simulink model "Attitude_Control_Pyramidal_Configuration"  (R2024b)
settings: Solver=VariableStepAuto  StartTime=0.0  StopTime=10.0  RelTol=1e-3
libraries: slpidlib x7, simulink_extras x1, matrix_library x1, aerolibutil x1
settings Model: Creator=LEGION  LastModifiedBy=LEGION
settings DebuggingCC: AlgebraicLoopMsg=none

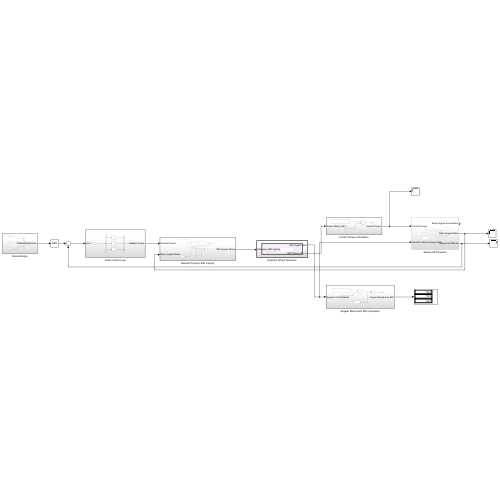
[thumbnail: Simulink's stored preview of the top-level diagram]
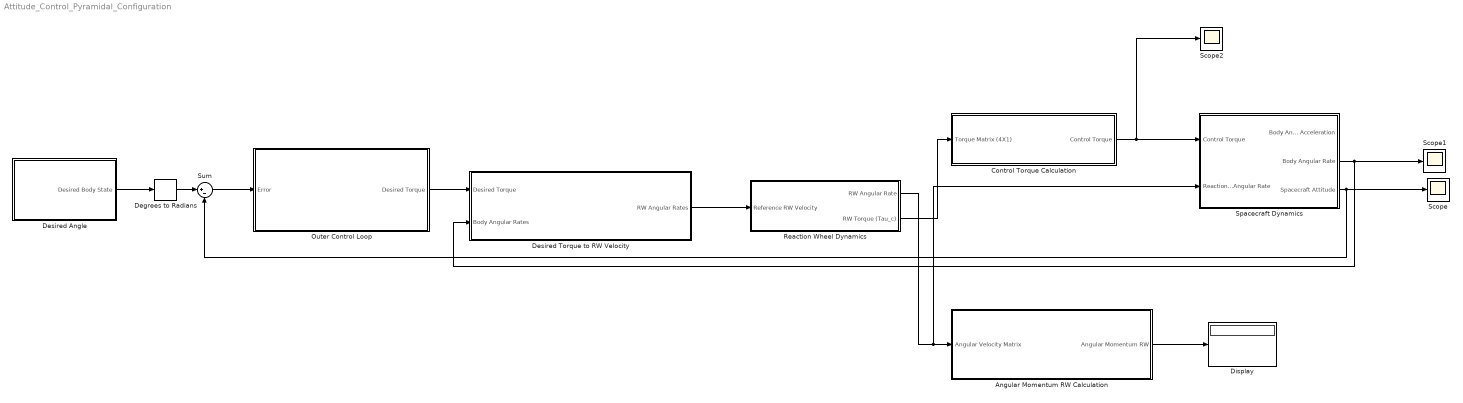
== system Attitude_Control_Pyramidal_Configuration ==
  Angular Momentum RW Calculation : Subsystem
  Control Torque Calculation : Subsystem
  Degrees to Radians : simulink_extras/Transformations/Degrees to Radians
  Desired Angle : Subsystem
  Desired Torque to RW Velocity : Subsystem
  Display : Display
  Outer Control Loop : Subsystem
  Reaction Wheel Dynamics : Subsystem  TreatAsAtomicUnit=on
      settings: MinAlgLoopOccurrences=on
  Scope : Scope
  Scope1 : Scope
  Scope2 : Scope
  Spacecraft Dynamics : Subsystem
      settings: PermitHierarchicalResolution=None  MinAlgLoopOccurrences=on
  Sum : Sum  Inputs=|+-
  wires:
  Control Torque Calculation/1(Control Torque) -> Scope2/1, Spacecraft Dynamics/1(Control Torque)
  Desired Angle/1(Desired Body State) -> Degrees to Radians/1
  Degrees to Radians/1 -> Sum/1
  Sum/1 -> Outer Control Loop/1(Error)
  Outer Control Loop/1(Desired Torque) -> Desired Torque to RW Velocity/1(Desired Torque)
  Reaction Wheel Dynamics/1(RW Angular Rate) -> Spacecraft Dynamics/2(Reaction Wheel Angular Rate), Angular Momentum RW Calculation/1("Angular Velocity Matrix ")
  Reaction Wheel Dynamics/2(RW Torque (Tau_c)) -> Control Torque Calculation/1(Torque Matrix (4X1))
  Desired Torque to RW Velocity/1(RW Angular Rates) -> Reaction Wheel Dynamics/1(Reference RW Velocity)
  Spacecraft Dynamics/2(Body Angular Rate) -> Scope1/1, Desired Torque to RW Velocity/2(Body Angular Rates)
  Spacecraft Dynamics/3(Spacecraft Attitude) -> Scope/1, Sum/2
  Angular Momentum RW Calculation/1(Angular Momentum RW) -> Display/1

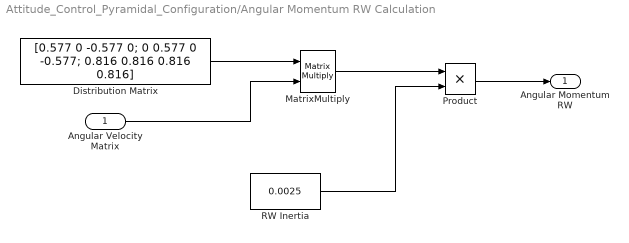
== system Attitude_Control_Pyramidal_Configuration/Angular Momentum RW Calculation ==
  "Angular Velocity Matrix " : Inport
  Distribution Matrix : Constant  Value=[0.577 0 -0.577 0; 0 0.577 0 -0.577; 0.816 0.816 0.816 0.816]  VectorParams1D=off
  MatrixMultiply : Product  Multiplication=Matrix(*)
  Product : Product
  RW Inertia : Constant  Value=0.0025
  Angular Momentum RW : Outport
  wires:
  Distribution Matrix/1 -> MatrixMultiply/1
  "Angular Velocity Matrix "/1 -> MatrixMultiply/2
  MatrixMultiply/1 -> Product/1
  RW Inertia/1 -> Product/2
  Product/1 -> Angular Momentum RW/1

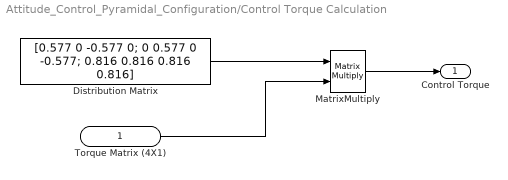
== system Attitude_Control_Pyramidal_Configuration/Control Torque Calculation ==
  Torque Matrix (4X1) : Inport
  Distribution Matrix : Constant  Value=[0.577 0 -0.577 0; 0 0.577 0 -0.577; 0.816 0.816 0.816 0.816]  VectorParams1D=off
  MatrixMultiply : Product  Multiplication=Matrix(*)
  Control Torque : Outport
  wires:
  Distribution Matrix/1 -> MatrixMultiply/1
  Torque Matrix (4X1)/1 -> MatrixMultiply/2
  MatrixMultiply/1 -> Control Torque/1

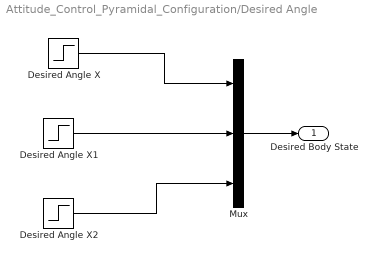
== system Attitude_Control_Pyramidal_Configuration/Desired Angle ==
  Desired Angle X : Step  Time=0.1  After=90  SampleTime=0  VectorParams1D=off
  Desired Angle X1 : Step  Time=0.1  After=90  SampleTime=0  VectorParams1D=off
  Desired Angle X2 : Step  Time=0.1  After=90  SampleTime=0  VectorParams1D=off
  Mux : Mux  Inputs=3
  Desired Body State : Outport
  wires:
  Desired Angle X1/1 -> Mux/2
  Desired Angle X/1 -> Mux/1
  Desired Angle X2/1 -> Mux/3
  Mux/1 -> Desired Body State/1

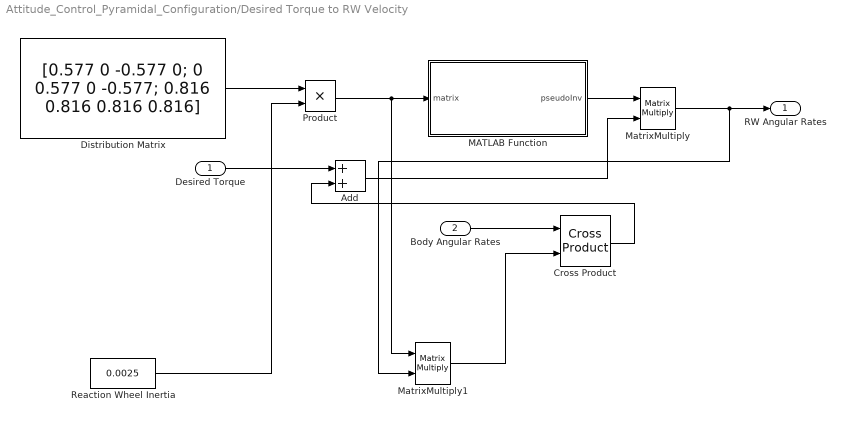
== system Attitude_Control_Pyramidal_Configuration/Desired Torque to RW Velocity ==
  Desired Torque : Inport
  Body Angular Rates : Inport  Port=2
  Add : Sum
  Cross Product : matrix_library/Cross Product
  Distribution Matrix : Constant  Value=[0.577 0 -0.577 0; 0 0.577 0 -0.577; 0.816 0.816 0.816 0.816]  VectorParams1D=off
  MATLAB Function : MATLAB Function  TreatAsAtomicUnit=on
  MatrixMultiply : Product  Multiplication=Matrix(*)
  MatrixMultiply1 : Product  Multiplication=Matrix(*)
  Product : Product
  Reaction Wheel Inertia : Constant  Value=0.0025
  RW Angular Rates : Outport
  wires:
  Desired Torque/1 -> Add/1
  Distribution Matrix/1 -> Product/1
  Reaction Wheel Inertia/1 -> Product/2
  Product/1 -> MATLAB Function/1(matrix), MatrixMultiply1/1
  MATLAB Function/1(pseudoInv) -> MatrixMultiply/1
  Body Angular Rates/1 -> Cross Product/1
  Cross Product/1 -> Add/2
  Add/1 -> MatrixMultiply/2
  MatrixMultiply/1 -> MatrixMultiply1/2, RW Angular Rates/1
  MatrixMultiply1/1 -> Cross Product/2

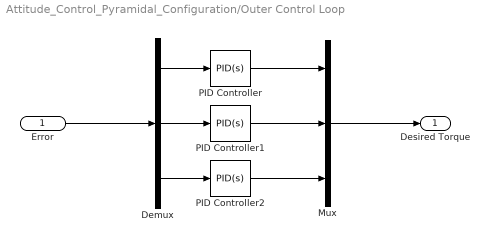
== system Attitude_Control_Pyramidal_Configuration/Outer Control Loop ==
  Error : Inport
  Demux : Demux  Outputs=3
  Mux : Mux  Inputs=3
  PID Controller : slpidlib/PID Controller  Controller=PID  Form=Parallel  TimeDomain=Continuous-time  UseExternalTs=off  SampleTime=-1  IntegratorMethod=Forward Euler  FilterMethod=Forward Euler  ControllerParametersSource=internal  P=100  I=1  UseKiTs=off  D=5  UseExternalDerivativeSource=off  N=100  UseFilter=on  TunerSelectOption=Transfer Function Based (PID Tuner App)  InitialConditionSource=internal  InitialConditionForIntegrator=0  InitialConditionForFilter=0  DifferentiatorICPrevScaledInput=0  ExternalReset=none  TrackingMode=off  Kt=1  LimitOutput=off  SatLimitsSource=internal  UpperSaturationLimit=inf  LowerSaturationLimit=-inf  LinearizeAsGain=on  AntiWindupMode=none  Kb=1  LimitIntegrator=off  UpperIntegratorSaturationLimit=inf  LowerIntegratorSaturationLimit=-inf  POutMin=[]  POutMax=[]  IOutMin=[]  IOutMax=[]  DOutMin=[]  DOutMax=[]  NOutMin=[]  NOutMax=[]  SumOutMin=[]  SumOutMax=[]  SaturationOutMin=[]  SaturationOutMax=[]  PParamMin=[]  PParamMax=[]  IParamMin=[]  IParamMax=[]  DParamMin=[]  DParamMax=[]  NParamMin=[]  NParamMax=[]  KbParamMin=[]  KbParamMax=[]  KtParamMin=[]  KtParamMax=[]  KbOutMin=[]  KbOutMax=[]  KtOutMin=[]  KtOutMax=[]  IntegratorOutMin=[]  IntegratorOutMax=[]  FilterOutMin=[]  FilterOutMax=[]  SumI1OutMin=[]  SumI1OutMax=[]  SumI2OutMin=[]  SumI2OutMax=[]  SumI3OutMin=[]  SumI3OutMax=[]  SumI4OutMin=[]  SumI4OutMax=[]  SumDOutMin=[]  SumDOutMax=[]  DifferentiatorOutMin=[]  DifferentiatorOutMax=[]  FilterDiffOutCoefMin=[]  FilterDiffOutCoefMax=[]  ReciprocalOutMin=[]  ReciprocalOutMax=[]  SumDenOutMin=[]  SumDenOutMax=[]  SumNumOutMin=[]  SumNumOutMax=[]  DivideOutMin=[]  DivideOutMax=[]  UdiffTsProdOutMin=[]  UdiffTsProdOutMax=[]  NTsProdOutMin=[]  NTsProdOutMax=[]  UintegralTsProdOutMin=[]  UintegralTsProdOutMax=[]  UngainTsProdOutMin=[]  UngainTsProdOutMax=[]  ClampingZeroOutDataTypeStr=Inherit: Inherit via back propagation  ClampingZeroOutMin=[]  ClampingZeroOutMax=[]  FilterDenConstantOutDataTypeStr=Inherit: Inherit via back propagation  FilterDenConstantOutMin=[]  FilterDenConstantOutMax=[]  PCopyOutDataTypeStr=Inherit: Inherit via back propagation  PCopyOutMin=[]  PCopyOutMax=[]  NCopyOutDataTypeStr=Inherit: Inherit via back propagation  NCopyOutMin=[]  NCopyOutMax=[]  IntegratorContinuousStateAttributes=''  IntegratorStateMustResolveToSignalObject=off  IntegratorRTWStateStorageClass=Auto  FilterContinuousStateAttributes=''  FilterStateMustResolveToSignalObject=off  FilterRTWStateStorageClass=Auto  ParallelPVariant=InternalParameters  IdealPVariant=Disabled  IVariant=InternalParameters  DVariant=InternalParameters  IntegratorVariant=Continuous  SatVariant=Disabled  AWVariant=Passthrough  PCopyVariant=Disabled  TRVariant=Disabled  FdbkBlocksVariant=Forward  IdealPFdbkVariant=Disabled  SatFdbkVariant=Disabled  DerivativeFilterVariant=ContFilter  NVariant=InternalParameters  NCopyVariant=Disabled  FilterICVariant=InternalICsFilter  IntegratorICVariant=InternalICs  ExternalResetVariant=Disabled  TRSumVariant=Passthrough  SumFdbkVariant=Disabled  SumVariant=Sum_PID  TsampFilterVariant=InternalTs  TsampNgainVariant=Passthrough  TsampIntegralVariant=Disabled_SignalSpec  ExternalSaturationOutDataTypeStr=Inherit: Same as second input  DerivativeSourceVariant=ErrorSignal  PreIntVariant=InternalPreInt
  PID Controller1 : slpidlib/PID Controller  Controller=PID  Form=Parallel  TimeDomain=Continuous-time  UseExternalTs=off  SampleTime=-1  IntegratorMethod=Forward Euler  FilterMethod=Forward Euler  ControllerParametersSource=internal  P=100  I=1  UseKiTs=off  D=5  UseExternalDerivativeSource=off  N=100  UseFilter=on  TunerSelectOption=Transfer Function Based (PID Tuner App)  InitialConditionSource=internal  InitialConditionForIntegrator=0  InitialConditionForFilter=0  DifferentiatorICPrevScaledInput=0  ExternalReset=none  TrackingMode=off  Kt=1  LimitOutput=off  SatLimitsSource=internal  UpperSaturationLimit=inf  LowerSaturationLimit=-inf  LinearizeAsGain=on  AntiWindupMode=none  Kb=1  LimitIntegrator=off  UpperIntegratorSaturationLimit=inf  LowerIntegratorSaturationLimit=-inf  POutMin=[]  POutMax=[]  IOutMin=[]  IOutMax=[]  DOutMin=[]  DOutMax=[]  NOutMin=[]  NOutMax=[]  SumOutMin=[]  SumOutMax=[]  SaturationOutMin=[]  SaturationOutMax=[]  PParamMin=[]  PParamMax=[]  IParamMin=[]  IParamMax=[]  DParamMin=[]  DParamMax=[]  NParamMin=[]  NParamMax=[]  KbParamMin=[]  KbParamMax=[]  KtParamMin=[]  KtParamMax=[]  KbOutMin=[]  KbOutMax=[]  KtOutMin=[]  KtOutMax=[]  IntegratorOutMin=[]  IntegratorOutMax=[]  FilterOutMin=[]  FilterOutMax=[]  SumI1OutMin=[]  SumI1OutMax=[]  SumI2OutMin=[]  SumI2OutMax=[]  SumI3OutMin=[]  SumI3OutMax=[]  SumI4OutMin=[]  SumI4OutMax=[]  SumDOutMin=[]  SumDOutMax=[]  DifferentiatorOutMin=[]  DifferentiatorOutMax=[]  FilterDiffOutCoefMin=[]  FilterDiffOutCoefMax=[]  ReciprocalOutMin=[]  ReciprocalOutMax=[]  SumDenOutMin=[]  SumDenOutMax=[]  SumNumOutMin=[]  SumNumOutMax=[]  DivideOutMin=[]  DivideOutMax=[]  UdiffTsProdOutMin=[]  UdiffTsProdOutMax=[]  NTsProdOutMin=[]  NTsProdOutMax=[]  UintegralTsProdOutMin=[]  UintegralTsProdOutMax=[]  UngainTsProdOutMin=[]  UngainTsProdOutMax=[]  ClampingZeroOutDataTypeStr=Inherit: Inherit via back propagation  ClampingZeroOutMin=[]  ClampingZeroOutMax=[]  FilterDenConstantOutDataTypeStr=Inherit: Inherit via back propagation  FilterDenConstantOutMin=[]  FilterDenConstantOutMax=[]  PCopyOutDataTypeStr=Inherit: Inherit via back propagation  PCopyOutMin=[]  PCopyOutMax=[]  NCopyOutDataTypeStr=Inherit: Inherit via back propagation  NCopyOutMin=[]  NCopyOutMax=[]  IntegratorContinuousStateAttributes=''  IntegratorStateMustResolveToSignalObject=off  IntegratorRTWStateStorageClass=Auto  FilterContinuousStateAttributes=''  FilterStateMustResolveToSignalObject=off  FilterRTWStateStorageClass=Auto  ParallelPVariant=InternalParameters  IdealPVariant=Disabled  IVariant=InternalParameters  DVariant=InternalParameters  IntegratorVariant=Continuous  SatVariant=Disabled  AWVariant=Passthrough  PCopyVariant=Disabled  TRVariant=Disabled  FdbkBlocksVariant=Forward  IdealPFdbkVariant=Disabled  SatFdbkVariant=Disabled  DerivativeFilterVariant=ContFilter  NVariant=InternalParameters  NCopyVariant=Disabled  FilterICVariant=InternalICsFilter  IntegratorICVariant=InternalICs  ExternalResetVariant=Disabled  TRSumVariant=Passthrough  SumFdbkVariant=Disabled  SumVariant=Sum_PID  TsampFilterVariant=InternalTs  TsampNgainVariant=Passthrough  TsampIntegralVariant=Disabled_SignalSpec  ExternalSaturationOutDataTypeStr=Inherit: Same as second input  DerivativeSourceVariant=ErrorSignal  PreIntVariant=InternalPreInt
  PID Controller2 : slpidlib/PID Controller  Controller=PID  Form=Parallel  TimeDomain=Continuous-time  UseExternalTs=off  SampleTime=-1  IntegratorMethod=Forward Euler  FilterMethod=Forward Euler  ControllerParametersSource=internal  P=100  I=1  UseKiTs=off  D=5  UseExternalDerivativeSource=off  N=100  UseFilter=on  TunerSelectOption=Transfer Function Based (PID Tuner App)  InitialConditionSource=internal  InitialConditionForIntegrator=0  InitialConditionForFilter=0  DifferentiatorICPrevScaledInput=0  ExternalReset=none  TrackingMode=off  Kt=1  LimitOutput=off  SatLimitsSource=internal  UpperSaturationLimit=inf  LowerSaturationLimit=-inf  LinearizeAsGain=on  AntiWindupMode=none  Kb=1  LimitIntegrator=off  UpperIntegratorSaturationLimit=inf  LowerIntegratorSaturationLimit=-inf  POutMin=[]  POutMax=[]  IOutMin=[]  IOutMax=[]  DOutMin=[]  DOutMax=[]  NOutMin=[]  NOutMax=[]  SumOutMin=[]  SumOutMax=[]  SaturationOutMin=[]  SaturationOutMax=[]  PParamMin=[]  PParamMax=[]  IParamMin=[]  IParamMax=[]  DParamMin=[]  DParamMax=[]  NParamMin=[]  NParamMax=[]  KbParamMin=[]  KbParamMax=[]  KtParamMin=[]  KtParamMax=[]  KbOutMin=[]  KbOutMax=[]  KtOutMin=[]  KtOutMax=[]  IntegratorOutMin=[]  IntegratorOutMax=[]  FilterOutMin=[]  FilterOutMax=[]  SumI1OutMin=[]  SumI1OutMax=[]  SumI2OutMin=[]  SumI2OutMax=[]  SumI3OutMin=[]  SumI3OutMax=[]  SumI4OutMin=[]  SumI4OutMax=[]  SumDOutMin=[]  SumDOutMax=[]  DifferentiatorOutMin=[]  DifferentiatorOutMax=[]  FilterDiffOutCoefMin=[]  FilterDiffOutCoefMax=[]  ReciprocalOutMin=[]  ReciprocalOutMax=[]  SumDenOutMin=[]  SumDenOutMax=[]  SumNumOutMin=[]  SumNumOutMax=[]  DivideOutMin=[]  DivideOutMax=[]  UdiffTsProdOutMin=[]  UdiffTsProdOutMax=[]  NTsProdOutMin=[]  NTsProdOutMax=[]  UintegralTsProdOutMin=[]  UintegralTsProdOutMax=[]  UngainTsProdOutMin=[]  UngainTsProdOutMax=[]  ClampingZeroOutDataTypeStr=Inherit: Inherit via back propagation  ClampingZeroOutMin=[]  ClampingZeroOutMax=[]  FilterDenConstantOutDataTypeStr=Inherit: Inherit via back propagation  FilterDenConstantOutMin=[]  FilterDenConstantOutMax=[]  PCopyOutDataTypeStr=Inherit: Inherit via back propagation  PCopyOutMin=[]  PCopyOutMax=[]  NCopyOutDataTypeStr=Inherit: Inherit via back propagation  NCopyOutMin=[]  NCopyOutMax=[]  IntegratorContinuousStateAttributes=''  IntegratorStateMustResolveToSignalObject=off  IntegratorRTWStateStorageClass=Auto  FilterContinuousStateAttributes=''  FilterStateMustResolveToSignalObject=off  FilterRTWStateStorageClass=Auto  ParallelPVariant=InternalParameters  IdealPVariant=Disabled  IVariant=InternalParameters  DVariant=InternalParameters  IntegratorVariant=Continuous  SatVariant=Disabled  AWVariant=Passthrough  PCopyVariant=Disabled  TRVariant=Disabled  FdbkBlocksVariant=Forward  IdealPFdbkVariant=Disabled  SatFdbkVariant=Disabled  DerivativeFilterVariant=ContFilter  NVariant=InternalParameters  NCopyVariant=Disabled  FilterICVariant=InternalICsFilter  IntegratorICVariant=InternalICs  ExternalResetVariant=Disabled  TRSumVariant=Passthrough  SumFdbkVariant=Disabled  SumVariant=Sum_PID  TsampFilterVariant=InternalTs  TsampNgainVariant=Passthrough  TsampIntegralVariant=Disabled_SignalSpec  ExternalSaturationOutDataTypeStr=Inherit: Same as second input  DerivativeSourceVariant=ErrorSignal  PreIntVariant=InternalPreInt
  Desired Torque : Outport
  wires:
  Error/1 -> Demux/1
  Demux/1 -> PID Controller/1
  Demux/2 -> PID Controller1/1
  Demux/3 -> PID Controller2/1
  PID Controller/1 -> Mux/1
  PID Controller1/1 -> Mux/2
  PID Controller2/1 -> Mux/3
  Mux/1 -> Desired Torque/1

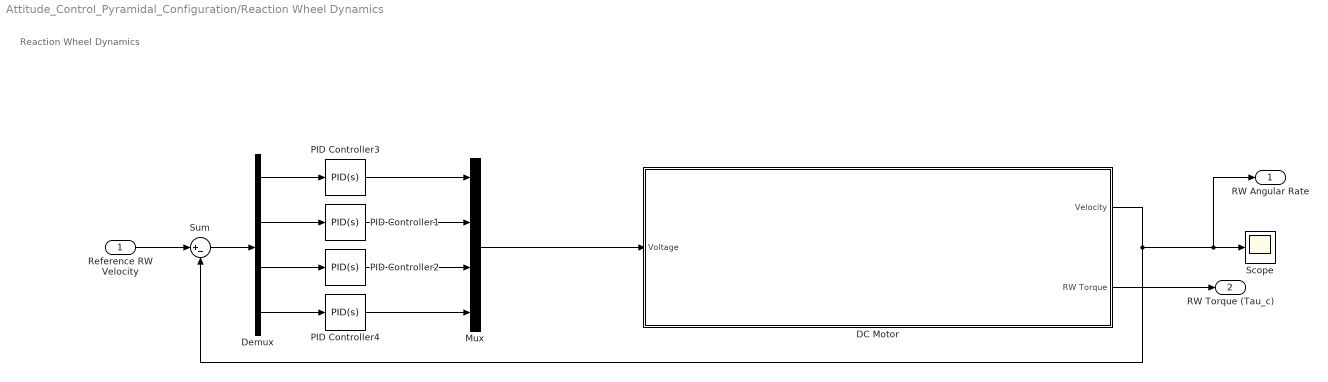
== system Attitude_Control_Pyramidal_Configuration/Reaction Wheel Dynamics ==
  note: Reaction Wheel Dynamics
  Reference RW Velocity : Inport
  "DC Motor " : Subsystem
  Demux : Demux
  Mux : Mux
  PID Controller{1..4} (4 alike) : slpidlib/PID Controller  Controller=PID  Form=Parallel  TimeDomain=Continuous-time  UseExternalTs=off  SampleTime=-1  IntegratorMethod=Forward Euler  FilterMethod=Forward Euler  ControllerParametersSource=internal  P=0.0171217142145511  I=12.0565982426295  UseKiTs=off  D=0  UseExternalDerivativeSource=off  N=100  UseFilter=on  TunerSelectOption=Transfer Function Based (PID Tuner App)  InitialConditionSource=internal  InitialConditionForIntegrator=0  InitialConditionForFilter=0  DifferentiatorICPrevScaledInput=0  ExternalReset=none  TrackingMode=off  Kt=1  LimitOutput=off  SatLimitsSource=internal  UpperSaturationLimit=inf  LowerSaturationLimit=-inf  LinearizeAsGain=on  AntiWindupMode=none  Kb=1  LimitIntegrator=off  UpperIntegratorSaturationLimit=inf  LowerIntegratorSaturationLimit=-inf  POutMin=[]  POutMax=[]  IOutMin=[]  IOutMax=[]  DOutMin=[]  DOutMax=[]  NOutMin=[]  NOutMax=[]  SumOutMin=[]  SumOutMax=[]  SaturationOutMin=[]  SaturationOutMax=[]  PParamMin=[]  PParamMax=[]  IParamMin=[]  IParamMax=[]  DParamMin=[]  DParamMax=[]  NParamMin=[]  NParamMax=[]  KbParamMin=[]  KbParamMax=[]  KtParamMin=[]  KtParamMax=[]  KbOutMin=[]  KbOutMax=[]  KtOutMin=[]  KtOutMax=[]  IntegratorOutMin=[]  IntegratorOutMax=[]  FilterOutMin=[]  FilterOutMax=[]  SumI1OutMin=[]  SumI1OutMax=[]  SumI2OutMin=[]  SumI2OutMax=[]  SumI3OutMin=[]  SumI3OutMax=[]  SumI4OutMin=[]  SumI4OutMax=[]  SumDOutMin=[]  SumDOutMax=[]  DifferentiatorOutMin=[]  DifferentiatorOutMax=[]  FilterDiffOutCoefMin=[]  FilterDiffOutCoefMax=[]  ReciprocalOutMin=[]  ReciprocalOutMax=[]  SumDenOutMin=[]  SumDenOutMax=[]  SumNumOutMin=[]  SumNumOutMax=[]  DivideOutMin=[]  DivideOutMax=[]  UdiffTsProdOutMin=[]  UdiffTsProdOutMax=[]  NTsProdOutMin=[]  NTsProdOutMax=[]  UintegralTsProdOutMin=[]  UintegralTsProdOutMax=[]  UngainTsProdOutMin=[]  UngainTsProdOutMax=[]  ClampingZeroOutDataTypeStr=Inherit: Inherit via back propagation  ClampingZeroOutMin=[]  ClampingZeroOutMax=[]  FilterDenConstantOutDataTypeStr=Inherit: Inherit via back propagation  FilterDenConstantOutMin=[]  FilterDenConstantOutMax=[]  PCopyOutDataTypeStr=Inherit: Inherit via back propagation  PCopyOutMin=[]  PCopyOutMax=[]  NCopyOutDataTypeStr=Inherit: Inherit via back propagation  NCopyOutMin=[]  NCopyOutMax=[]  IntegratorContinuousStateAttributes=''  IntegratorStateMustResolveToSignalObject=off  IntegratorRTWStateStorageClass=Auto  FilterContinuousStateAttributes=''  FilterStateMustResolveToSignalObject=off  FilterRTWStateStorageClass=Auto  ParallelPVariant=InternalParameters  IdealPVariant=Disabled  IVariant=InternalParameters  DVariant=InternalParameters  IntegratorVariant=Continuous  SatVariant=Disabled  AWVariant=Passthrough  PCopyVariant=Disabled  TRVariant=Disabled  FdbkBlocksVariant=Forward  IdealPFdbkVariant=Disabled  SatFdbkVariant=Disabled  DerivativeFilterVariant=ContFilter  NVariant=InternalParameters  NCopyVariant=Disabled  FilterICVariant=InternalICsFilter  IntegratorICVariant=InternalICs  ExternalResetVariant=Disabled  TRSumVariant=Passthrough  SumFdbkVariant=Disabled  SumVariant=Sum_PID  TsampFilterVariant=InternalTs  TsampNgainVariant=Passthrough  TsampIntegralVariant=Disabled_SignalSpec  ExternalSaturationOutDataTypeStr=Inherit: Same as second input  DerivativeSourceVariant=ErrorSignal  PreIntVariant=InternalPreInt
  Scope : Scope
  Sum : Sum  Inputs=|+-
  RW Angular Rate : Outport
  RW Torque (Tau_c) : Outport  Port=2
  wires:
  "DC Motor "/1(Velocity) -> Sum/2, RW Angular Rate/1, Scope/1
  Sum/1 -> Demux/1
  Demux/1 -> PID Controller3/1
  PID Controller2/1 -> Mux/3
  PID Controller1/1 -> Mux/2
  Mux/1 -> "DC Motor "/1(Voltage)
  Demux/3 -> PID Controller2/1
  PID Controller3/1 -> Mux/1
  Demux/2 -> PID Controller1/1
  Reference RW Velocity/1 -> Sum/1
  Demux/4 -> PID Controller4/1
  PID Controller4/1 -> Mux/4
  "DC Motor "/2(RW Torque) -> RW Torque (Tau_c)/1

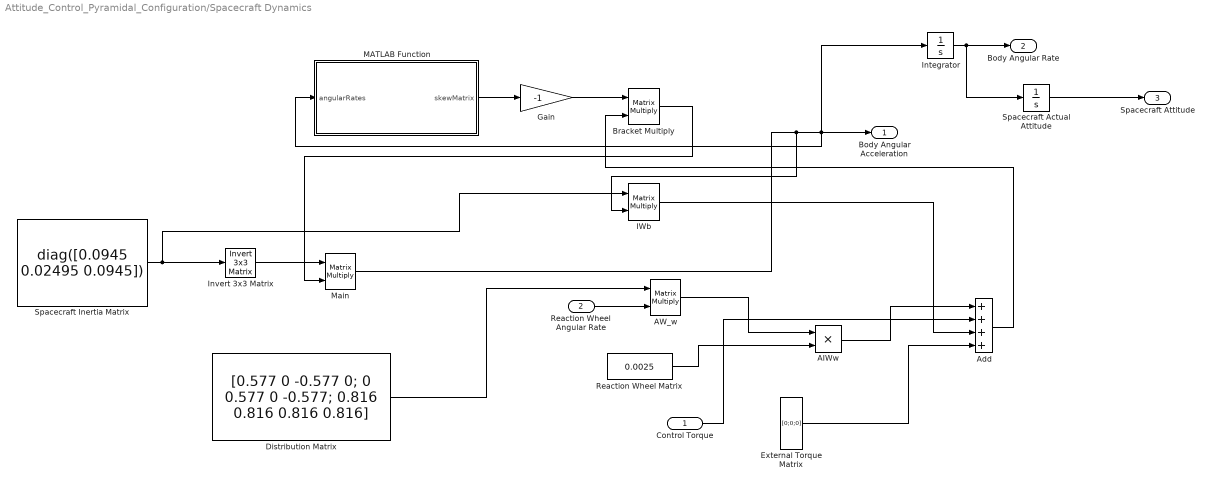
== system Attitude_Control_Pyramidal_Configuration/Spacecraft Dynamics ==
  Control Torque : Inport
  Reaction Wheel Angular Rate : Inport  Port=2
  AIWw : Product
  AW_w : Product  Multiplication=Matrix(*)
  Add : Sum  Inputs=++++
  Bracket Multiply : Product  Multiplication=Matrix(*)
  Distribution Matrix : Constant  Value=[0.577 0 -0.577 0; 0 0.577 0 -0.577; 0.816 0.816 0.816 0.816]  VectorParams1D=off
  External Torque Matrix : Constant  Value=[0;0;0]  VectorParams1D=off
  Gain : Gain  Gain=-1
  IWb : Product  Multiplication=Matrix(*)
  Integrator : Integrator
  Invert 3x3 Matrix : aerolibutil/Invert  3x3 Matrix
  MATLAB Function : MATLAB Function  TreatAsAtomicUnit=on
  Main : Product  Multiplication=Matrix(*)
  Reaction Wheel Matrix : Constant  Value=0.0025
  Spacecraft Actual Attitude : Integrator
  "Spacecraft Inertia Matrix " : Constant  Value=diag([0.0945 0.02495 0.0945])  VectorParams1D=off
  Body Angular Acceleration : Outport
  Body Angular Rate : Outport  Port=2
  Spacecraft Attitude : Outport  Port=3
  wires:
  "Spacecraft Inertia Matrix "/1 -> IWb/1, Invert 3x3 Matrix/1
  Invert 3x3 Matrix/1 -> Main/1
  MATLAB Function/1(skewMatrix) -> Gain/1
  Gain/1 -> Bracket Multiply/1
  Distribution Matrix/1 -> AW_w/1
  Reaction Wheel Angular Rate/1 -> AW_w/2
  AW_w/1 -> AIWw/1
  Reaction Wheel Matrix/1 -> AIWw/2
  AIWw/1 -> Add/1
  Control Torque/1 -> Add/2
  IWb/1 -> Add/3
  External Torque Matrix/1 -> Add/4
  Add/1 -> Bracket Multiply/2
  Bracket Multiply/1 -> Main/2
  Main/1 -> IWb/2, Integrator/1, MATLAB Function/1(angularRates), Body Angular Acceleration/1
  Integrator/1 -> Spacecraft Actual Attitude/1, Body Angular Rate/1
  Spacecraft Actual Attitude/1 -> Spacecraft Attitude/1

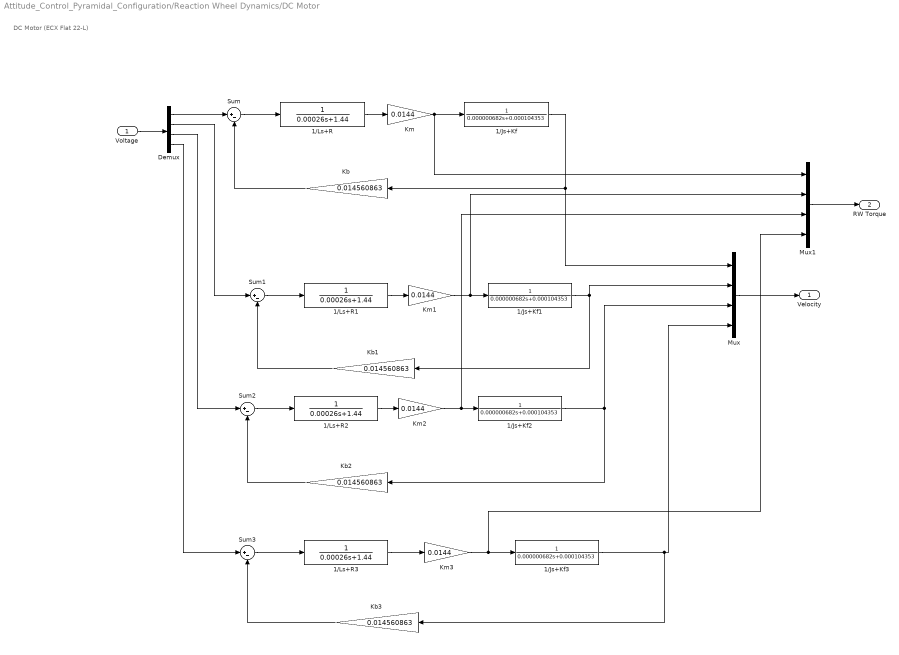
== system Attitude_Control_Pyramidal_Configuration/Reaction Wheel Dynamics/DC Motor  ==
  note: DC Motor (ECX Flat 22-L)
  Voltage : Inport
  1/Js+Kf{,1..3} (4 alike) : TransferFcn  Denominator=[0.000000682 0.000104353]
  1/Ls+R{,1..3} (4 alike) : TransferFcn  Denominator=[0.00026 1.44]
  Demux : Demux
  Kb{,1..3} (4 alike) : Gain  Gain=0.014560863
  Km{,1..3} (4 alike) : Gain  Gain=0.0144
  Mux : Mux  Inputs=4'
  Mux1 : Mux  Inputs=4'
  Sum{,1..3} (4 alike) : Sum  Inputs=|+-
  Velocity : Outport
  RW Torque : Outport  Port=2
  wires:
  Sum/1 -> 1/Ls+R/1
  1/Ls+R/1 -> Km/1
  Km/1 -> Mux1/1, 1/Js+Kf/1
  Kb/1 -> Sum/2
  Voltage/1 -> Demux/1
  Demux/1 -> Sum/1
  Km1/1 -> Mux1/2, 1/Js+Kf1/1
  Demux/2 -> Sum1/1
  Kb1/1 -> Sum1/2
  1/Ls+R1/1 -> Km1/1
  1/Js+Kf1/1 -> Kb1/1, Mux/2
  Sum1/1 -> 1/Ls+R1/1
  Km2/1 -> Mux1/3, 1/Js+Kf2/1
  Demux/3 -> Sum2/1
  1/Ls+R2/1 -> Km2/1
  1/Js+Kf2/1 -> Kb2/1, Mux/3
  Sum2/1 -> 1/Ls+R2/1
  1/Js+Kf/1 -> Kb/1, Mux/1
  Mux/1 -> Velocity/1
  Kb2/1 -> Sum2/2
  Demux/4 -> Sum3/1
  Sum3/1 -> 1/Ls+R3/1
  1/Js+Kf3/1 -> Kb3/1, Mux/4
  Km3/1 -> Mux1/4, 1/Js+Kf3/1
  1/Ls+R3/1 -> Km3/1
  Kb3/1 -> Sum3/2
  Mux1/1 -> RW Torque/1

== matlab function Attitude_Control_Pyramidal_Configuration/Spacecraft Dynamics/MATLAB Function ==
  data: angularRates input; skewMatrix output
function skewMatrix = angularRateSkew(angularRates)
    % Function to compute the skew-symmetric matrix for body angular rates
    % Input:
    %   angularRates - A 3x1 column vector [p; q; r]
    %                  where p, q, r are angular rates in rad/s
    % Output:
    %   skewMatrix - The 3x3 skew-symmetric matrix
    
    % Check if the input is a 3x1 vector
    if size(angularRates, 1) ~= 3 || size(angularRates, 2) ~= 1
        error('Input must be a 3x1 column vector representing angular rates.');
    end

    % Extract angular rate components
    p = angularRates(1); % Roll rate
    q = angularRates(2); % Pitch rate
    r = angularRates(3); % Yaw rate

    % Construct the skew-symmetric matrix
    skewMatrix = [  0, -r,  q;
                    r,  0, -p;
                   -q,  p,  0];
end

== matlab function Attitude_Control_Pyramidal_Configuration/Desired Torque to RW Velocity/MATLAB Function ==
  data: matrix input; pseudoInv output
function pseudoInv = invert3x4(matrix)
    % Function to compute the pseudo-inverse of a 3x4 matrix
    % Input:
    %   matrix - A 3x4 matrix
    % Output:
    %   pseudoInv - The pseudo-inverse of the input matrix
    
    % Check if the input is a 3x4 matrix
    if size(matrix, 1) ~= 3 || size(matrix, 2) ~= 4
        error('Input must be a 3x4 matrix.');
    end

    % Compute the pseudo-inverse
    pseudoInv = pinv(matrix);
end
